simulink model "Single_Phase_Grid_Connected_Converter"  (R2023b)
settings: Solver=VariableStepAuto  StartTime=0.0  StopTime=0.9  RelTol=1e-3
libraries: spsSeriesRLCBranchLib x4, spsCurrentMeasurementLib x2, spsVoltageMeasurementLib x2, spsDiodeLib x1, spsIGBTDiodeLib x1, slpidlib x1, spsPVArrayLib x1, spsPWMGeneratorDCDCLib x1, sps_lib x1
settings Model: Creator=aoni5  LastModifiedBy=aoni5

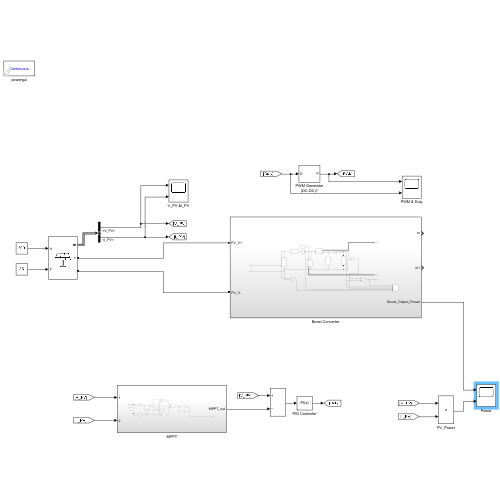
[thumbnail: Simulink's stored preview of the top-level diagram]
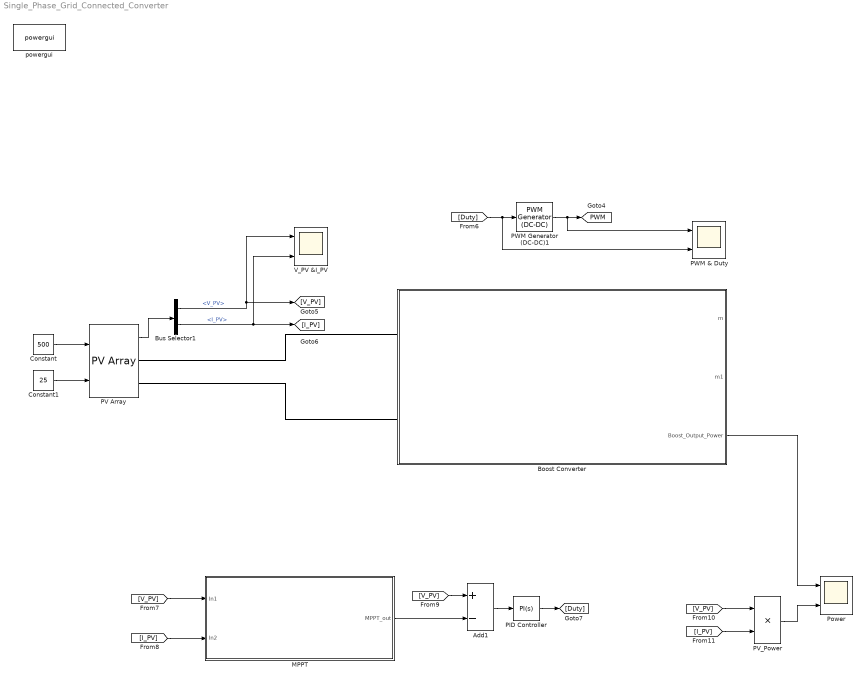
== system Single_Phase_Grid_Connected_Converter ==
  Add1 : Sum  Inputs=+-
  Boost Converter : Subsystem
  Bus Selector1 : BusSelector  OutputSignals=V_PV,I_PV
  Constant : Constant  Value=500
  Constant1 : Constant  Value=25
  MPPT : Subsystem
  PID Controller : slpidlib/PID Controller  Controller=PI  Form=Parallel  TimeDomain=Continuous-time  UseExternalTs=off  SampleTime=-1  IntegratorMethod=Forward Euler  FilterMethod=Forward Euler  ControllerParametersSource=internal  P=1  I=1  UseKiTs=off  D=0  N=100  UseFilter=on  TunerSelectOption=Transfer Function Based (PID Tuner App)  InitialConditionSource=internal  InitialConditionForIntegrator=0  InitialConditionForFilter=0  DifferentiatorICPrevScaledInput=0  ExternalReset=none  TrackingMode=off  Kt=1  LimitOutput=off  SatLimitsSource=internal  UpperSaturationLimit=inf  LowerSaturationLimit=-inf  LinearizeAsGain=on  AntiWindupMode=none  Kb=1  LimitIntegrator=off  UpperIntegratorSaturationLimit=inf  LowerIntegratorSaturationLimit=-inf  POutMin=[]  POutMax=[]  IOutMin=[]  IOutMax=[]  DOutMin=[]  DOutMax=[]  NOutMin=[]  NOutMax=[]  SumOutMin=[]  SumOutMax=[]  SaturationOutMin=[]  SaturationOutMax=[]  PParamMin=[]  PParamMax=[]  IParamMin=[]  IParamMax=[]  DParamMin=[]  DParamMax=[]  NParamMin=[]  NParamMax=[]  KbParamMin=[]  KbParamMax=[]  KtParamMin=[]  KtParamMax=[]  KbOutMin=[]  KbOutMax=[]  KtOutMin=[]  KtOutMax=[]  IntegratorOutMin=[]  IntegratorOutMax=[]  FilterOutMin=[]  FilterOutMax=[]  SumI1OutMin=[]  SumI1OutMax=[]  SumI2OutMin=[]  SumI2OutMax=[]  SumI3OutMin=[]  SumI3OutMax=[]  SumI4OutMin=[]  SumI4OutMax=[]  SumDOutMin=[]  SumDOutMax=[]  DifferentiatorOutMin=[]  DifferentiatorOutMax=[]  FilterDiffOutCoefMin=[]  FilterDiffOutCoefMax=[]  ReciprocalOutMin=[]  ReciprocalOutMax=[]  SumDenOutMin=[]  SumDenOutMax=[]  SumNumOutMin=[]  SumNumOutMax=[]  DivideOutMin=[]  DivideOutMax=[]  UdiffTsProdOutMin=[]  UdiffTsProdOutMax=[]  NTsProdOutMin=[]  NTsProdOutMax=[]  UintegralTsProdOutMin=[]  UintegralTsProdOutMax=[]  UngainTsProdOutMin=[]  UngainTsProdOutMax=[]  ClampingZeroOutDataTypeStr=Inherit: Inherit via back propagation  ClampingZeroOutMin=[]  ClampingZeroOutMax=[]  FilterDenConstantOutDataTypeStr=Inherit: Inherit via back propagation  FilterDenConstantOutMin=[]  FilterDenConstantOutMax=[]  PCopyOutDataTypeStr=Inherit: Inherit via back propagation  PCopyOutMin=[]  PCopyOutMax=[]  NCopyOutDataTypeStr=Inherit: Inherit via back propagation  NCopyOutMin=[]  NCopyOutMax=[]  IntegratorContinuousStateAttributes=''  IntegratorStateMustResolveToSignalObject=off  IntegratorRTWStateStorageClass=Auto  FilterContinuousStateAttributes=''  FilterStateMustResolveToSignalObject=off  FilterRTWStateStorageClass=Auto  ParallelPVariant=InternalParameters  IdealPVariant=Disabled  IVariant=InternalParameters  DVariant=Disabled  IntegratorVariant=Continuous  SatVariant=Disabled  AWVariant=Passthrough  PCopyVariant=Disabled  TRVariant=Disabled  FdbkBlocksVariant=Forward  IdealPFdbkVariant=Disabled  SatFdbkVariant=Disabled  DerivativeFilterVariant=Disabled  NVariant=Disabled  NCopyVariant=Disabled_SignalSpec  FilterICVariant=Disabled  IntegratorICVariant=InternalICs  ExternalResetVariant=Disabled  TRSumVariant=Passthrough  SumFdbkVariant=Disabled  SumVariant=Sum_PI  TsampFilterVariant=InternalTs  TsampNgainVariant=Passthrough  TsampIntegralVariant=Disabled_SignalSpec  ExternalSaturationOutDataTypeStr=Inherit: Same as second input
  PV Array : spsPVArrayLib/PV Array  Npar=2  Nser=3  PlotType=array @ 25 deg.C & specified irradiances  S_vec=[ 1000 800 600 400 200]  Temp_C_vec="[ 25  ]"  ModuleName=User-defined  PlotWhenSelected=off  Pm=314.1504  Ncell=81  Voc=81*0.727  Isc=6.45  Vm=0.640*81  Im=6.06  beta_Voc_pc=-1.74e-3/0.727*100  alpha_Isc_pc=2.9e-3/6.45*100  beta_Voc=-0.14094  alpha_Isc=0.0029  IL=6.4513  I0=1.3343e-12  nI=0.96977  Rsh=326.9714  Rs=0.064206  RobustModel=off  RobustCellTemperature=313.3991  BAL=on  Tc=1e-6  Tfilter=5e-5
  PV_Power : Product
  PWM & Duty : Scope  NumInputPorts=2
  PWM Generator (DC-DC)1 : spsPWMGeneratorDCDCLib/PWM Generator (DC-DC)  Fsw=7000  Ts=1e-6
  Power : Scope  NumInputPorts=2
  V_PV &I_PV : Scope  NumInputPorts=2
  powergui : sps_lib/powergui  Priority=1  SimulationMode=Continuous  SampleTime=50e-6  frequency=60  Iterations=50  frequencyindice=0  Pbase=100e6  ErrMax=1e-4  UnitsV=kV  UnitsW=MW  buscounter=0  FunctionMessages=off  echomessages=off  EnableUseOfTLC=off  CurrentSourceSwitches=off  DisableSnubberDevices=off  DisableRonSwitches=off  DisableVfSwitches=off  DisplayEquations=off  AutomaticDiscreteSolvers=off  SolverType=Tustin/Backward Euler (TBE)  Interpol=off  ExternalGateDelay=off  methode=off  Ts=100  x0status=blocks  SPID=on  SwTol=0  HookPort=off  NonlinearTolerance=1e-4  nMaxIteration=100  ContinueOnMaxIteration=off  RestoreLinks=warning  ResistiveCurrentMeasurement=off  Frange=[0:2:500]  Ylog=off  Xlog=on  ShowGrid=off  save=off  variable=ZData  structure=0  ZoomFFT=off  StartTime=0.0  cycles=1  DisplayStyle=1  fundamental=60  FreqAxis=off  MaxFrequency=1000  frequencyindicesteady=1  RmsSteady=1  display=off
  tag scope: PWM=global
  wires:
  [I_PV] -> MPPT/2(In2)
  MPPT/1(MPPT_out) -> Add1/2
  PV_Power/1 -> Power/2
  [V_PV] -> PV_Power/1
  [Duty] -> PWM & Duty/2, PWM Generator (DC-DC)1/1
  Bus Selector1/2 -> V_PV &I_PV/2, [I_PV]  "<I_PV>"
  Add1/1 -> PID Controller/1
  [V_PV] -> MPPT/1(In1)
  Bus Selector1/1 -> V_PV &I_PV/1, [V_PV]  "<V_PV>"
  [I_PV] -> PV_Power/2
  [V_PV] -> Add1/1
  Boost Converter/3(Boost_Output_Power) -> Power/1
  PID Controller/1 -> [Duty]
  PV Array/1 -> Bus Selector1/1
  PWM Generator (DC-DC)1/1 -> PWM & Duty/1, [PWM]
  Constant/1 -> PV Array/1
  Constant1/1 -> PV Array/2
  connections:
  Boost Converter/LConn2 -- PV Array/RConn2
  Boost Converter/LConn1 -- PV Array/RConn1

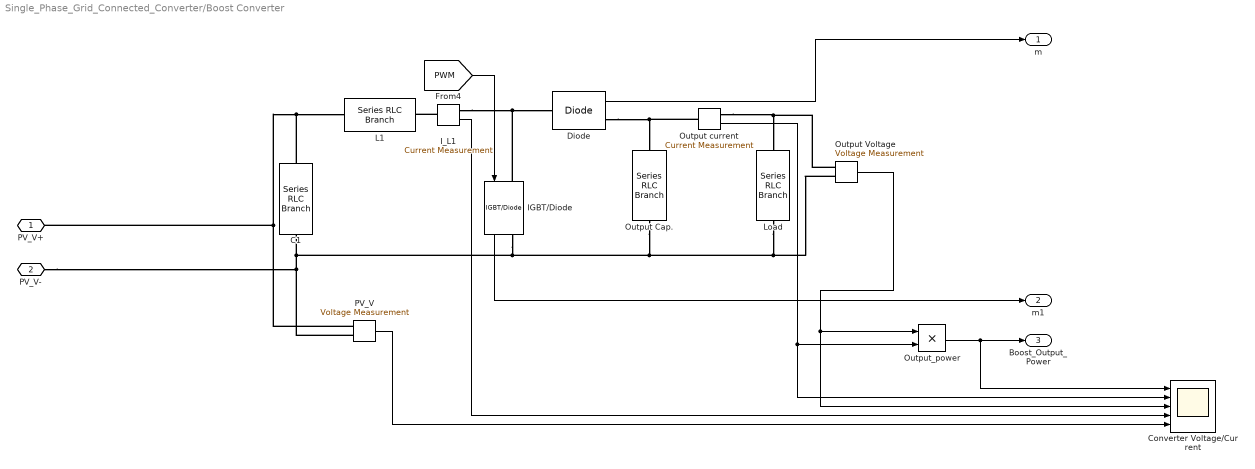
== system Single_Phase_Grid_Connected_Converter/Boost Converter ==
  C1 : spsSeriesRLCBranchLib/Series RLC Branch  LConnTagsString=__new0  RConnTagsString=__new0  BranchType=C  Resistance=1e-3  Inductance=1e-3  SetiL0=off  InitialCurrent=0  Capacitance=5500e-6  Setx0=off  InitialVoltage=0  Measurements=None
  Converter Voltage/Current : Scope  NumInputPorts=5
  Diode : spsDiodeLib/Diode  Ron=0.001  Lon=0  Vf=0.8  IC=0  UseSnubber=0  Rs=500  Cs=250e-9  Measurements=on
  IGBT/Diode : spsIGBTDiodeLib/IGBT//Diode  Ron=1e-3  Rs=1e5  Cs=inf  Measurements=on
  I_L1 : spsCurrentMeasurementLib/Current Measurement  PhasorSimulation=off  OutputType=Complex  PSBequivalent=0
  L1 : spsSeriesRLCBranchLib/Series RLC Branch  LConnTagsString=__new0  RConnTagsString=__new0  BranchType=L  Resistance=1e-3  Inductance=20e-3  SetiL0=off  InitialCurrent=0  Capacitance=1000e-6  Setx0=off  InitialVoltage=0  Measurements=None
  Load : spsSeriesRLCBranchLib/Series RLC Branch  LConnTagsString=__new0  RConnTagsString=__new0  BranchType=R  Resistance=48  Inductance=1e-3  SetiL0=off  InitialCurrent=0  Capacitance=5000e-6  Setx0=off  InitialVoltage=0  Measurements=None
  Output Cap. : spsSeriesRLCBranchLib/Series RLC Branch  LConnTagsString=__new0  RConnTagsString=__new0  BranchType=C  Resistance=1e-3  Inductance=1e-3  SetiL0=off  InitialCurrent=0  Capacitance=5500e-6  Setx0=off  InitialVoltage=0  Measurements=None
  Output Voltage : spsVoltageMeasurementLib/Voltage Measurement  PhasorSimulation=off  OutputType=Complex  PSBequivalent=0
  Output current : spsCurrentMeasurementLib/Current Measurement  PhasorSimulation=off  OutputType=Complex  PSBequivalent=0
  Output_power : Product
  PV_V : spsVoltageMeasurementLib/Voltage Measurement  PhasorSimulation=off  OutputType=Complex  PSBequivalent=0
  PV_V+ : PMIOPort  Side=Left
  PV_V- : PMIOPort  Port=2  Side=Left
  m : Outport
  m1 : Outport  Port=2
  Boost_Output_Power : Outport  Port=3
  wires:
  Output current/1 -> Output_power/2, Converter Voltage/Current/2
  Output Voltage/1 -> Converter Voltage/Current/3, Output_power/1
  I_L1/1 -> Converter Voltage/Current/4
  [PWM] -> IGBT/Diode/1
  PV_V/1 -> Converter Voltage/Current/5
  IGBT/Diode/1 -> m1/1
  Diode/1 -> m/1
  Output_power/1 -> Converter Voltage/Current/1, Boost_Output_Power/1
  connections:
  PV_V/LConn1 -- C1/RConn1 -- L1/LConn1 -- PV_V+/RConn1
  I_L1/RConn1 -- Diode/LConn1 -- IGBT/Diode/LConn1
  C1/LConn1 -- Output Voltage/LConn2 -- Load/RConn1 -- Output Cap./RConn1 -- IGBT/Diode/RConn1 -- PV_V/LConn2 -- PV_V-/RConn1
  Output current/LConn1 -- Output Cap./LConn1 -- Diode/RConn1
  Output Voltage/LConn1 -- Load/LConn1 -- Output current/RConn1
  I_L1/LConn1 -- L1/RConn1

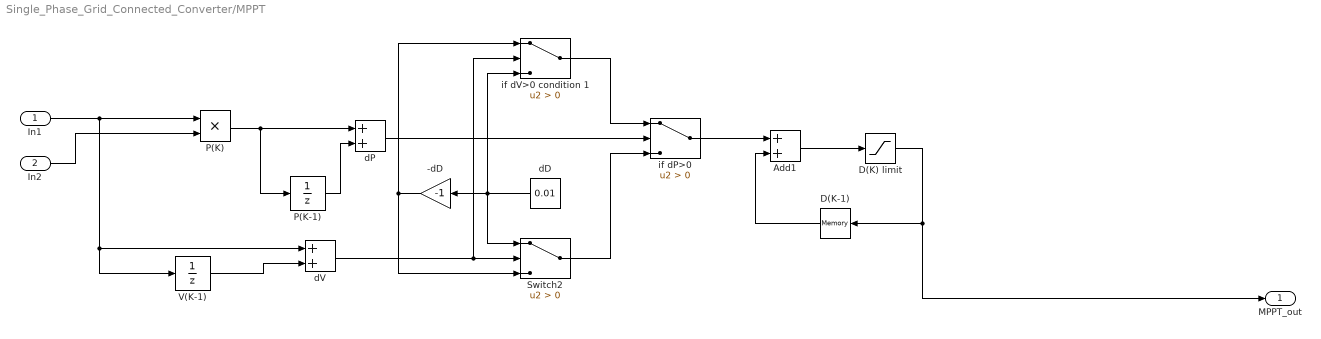
== system Single_Phase_Grid_Connected_Converter/MPPT ==
  In1 : Inport
  In2 : Inport  Port=2
  -dD : Gain  Gain=-1
  Add1 : Sum
  D(K) limit : Saturate  UpperLimit=160  LowerLimit=145
  D(K-1) : Memory
  P(K) : Product
  P(K-1) : UnitDelay  SampleTime=-1  HasFrameUpgradeWarning=on
  Switch2 : Switch  Criteria=u2 > Threshold  SaturateOnIntegerOverflow=off  InputSameDT=off
  V(K-1) : UnitDelay  SampleTime=-1  HasFrameUpgradeWarning=on
  dD : Constant  Value=0.01
  dP : Sum
  dV : Sum
  if dP>0 : Switch  Criteria=u2 > Threshold  SaturateOnIntegerOverflow=off  InputSameDT=off
  if dV>0 condition 1 : Switch  Criteria=u2 > Threshold  SaturateOnIntegerOverflow=off  InputSameDT=off
  MPPT_out : Outport
  wires:
  D(K) limit/1 -> MPPT_out/1, D(K-1)/1
  -dD/1 -> if dV>0 condition 1/1, Switch2/3
  dP/1 -> if dP>0/2
  P(K-1)/1 -> dP/2
  dD/1 -> if dV>0 condition 1/3, Switch2/1, -dD/1
  Switch2/1 -> if dP>0/3
  D(K-1)/1 -> Add1/2
  if dP>0/1 -> Add1/1
  In1/1 -> V(K-1)/1, dV/1, P(K)/1
  Add1/1 -> D(K) limit/1
  dV/1 -> Switch2/2, if dV>0 condition 1/2
  if dV>0 condition 1/1 -> if dP>0/1
  V(K-1)/1 -> dV/2
  P(K)/1 -> dP/1, P(K-1)/1
  In2/1 -> P(K)/2
